simulink model "propulsionMotorPrueba"  (R2016b)
settings: Solver=VariableStepAuto  StartTime=0.0  StopTime=10.0  RelTol=1e-3
undefined symbols (not defined in the file): LD, vms
libraries: simulink x1
settings Model: Creator=Uxío  LastModifiedBy=Uxío

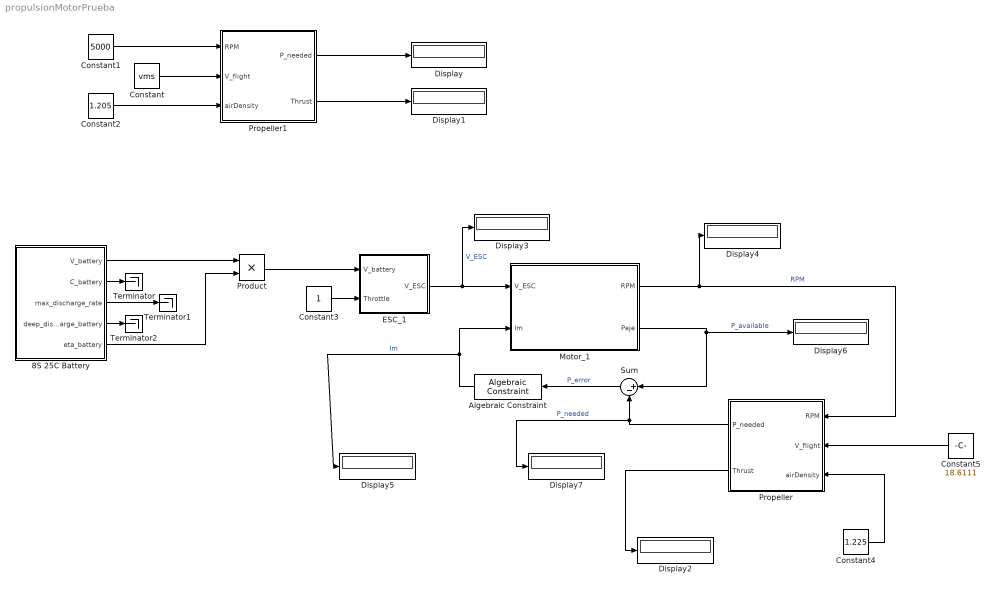
== system propulsionMotorPrueba ==
  8S 25C Battery : Subsystem
  Algebraic Constraint : simulink/Math Operations/Algebraic Constraint  z0=0
  Constant : Constant  Value=vms
  Constant1 : Constant  Value=5000
  Constant2 : Constant  Value=1.205
  Constant3 : Constant
  Constant4 : Constant  Value=1.225
  Constant5 : Constant  Value=18.6111
  Display{,1..7} (8 alike) : Display
  ESC_1 : Subsystem
  Motor_1 : Subsystem
  Product : Product
  Propeller : Subsystem
  Propeller1 : Subsystem
  Sum : Sum  Inputs=|+-
  Terminator : Terminator
  Terminator1 : Terminator
  Terminator2 : Terminator
  wires:
  Constant/1 -> Propeller1/2(V_flight)
  Constant1/1 -> Propeller1/1(RPM)
  Constant2/1 -> Propeller1/3(airDensity)
  Propeller1/1(P_needed) -> Display/1
  Propeller1/2(Thrust) -> Display1/1
  Constant3/1 -> ESC_1/2(Throttle)
  8S 25C Battery/1(V_battery) -> Product/1
  Product/1 -> ESC_1/1(V_battery)
  8S 25C Battery/5(eta_battery) -> Product/2
  8S 25C Battery/2(C_battery) -> Terminator/1
  8S 25C Battery/3(max_discharge_rate) -> Terminator1/1
  8S 25C Battery/4(deep_discharge_battery) -> Terminator2/1
  ESC_1/1(V_ESC) -> Motor_1/1(V_ESC), Display3/1  "V_ESC"
  Motor_1/1(RPM) -> Display4/1, Propeller/1(RPM)  "RPM"
  Constant5/1 -> Propeller/2(V_flight)
  Constant4/1 -> Propeller/3(airDensity)
  Propeller/1(P_needed) -> Display7/1, Sum/2  "P_needed"
  Motor_1/2(Peje) -> Display6/1, Sum/1  "P_available"
  Sum/1 -> Algebraic Constraint/1  "P_error"
  Algebraic Constraint/1 -> Motor_1/2(Im), Display5/1  "Im"
  Propeller/2(Thrust) -> Display2/1

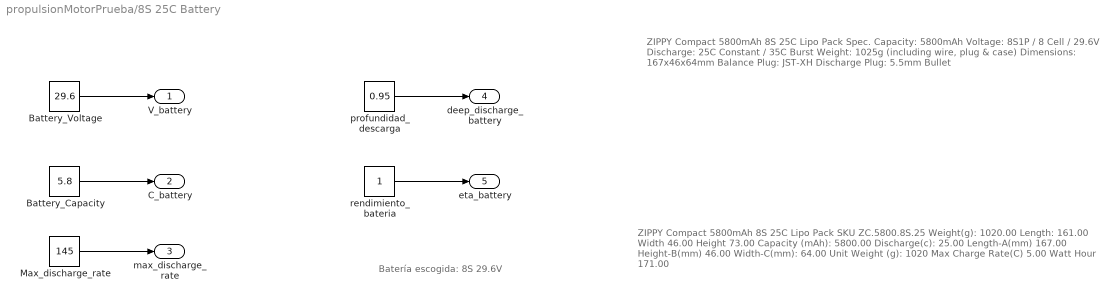
== system propulsionMotorPrueba/8S 25C Battery ==
  note: ZIPPY Compact 5800mAh 8S 25C Lipo Pack
      |
      | Spec.
      | Capacity: 5800mAh
      | Voltage: 8S1P / 8 Cell / 29.6V
      | Discharge: 25C Constant / 35C Burst
      | Weight: 1025g (including wire, plug & case)
      | Dimensions: 167x46x64mm
      | Balance Plug: JST-XH
      | Discharge Plug: 5.5mm Bullet
  note: ZIPPY Compact 5800mAh 8S 25C Lipo Pack
      |
      | SKU
      | ZC.5800.8S.25
      | Weight(g):
      | 1020.00
      | Length:
      | 161.00
      | Width
      | 46.00
      | Height
      | 73.00
      | Capacity (mAh):
      | 5800.00
      | Discharge(c):
      | 25.00
      | Length-A(mm)
      | 167.00
      | Height-B(mm)
      | 46.00
      | Width-C(mm):
      | 64.00
      | Unit Weight (g):
      | 1020
      | Max Charge Rate(C)
      | 5.00
      | Watt Hour
      | 171.00
  note: Batería escogida: 8S 29.6V
  Battery_Capacity : Constant  Value=5.8
  Battery_Voltage : Constant  Value=29.6
  Max_discharge_rate : Constant  Value=145
  profundidad_descarga : Constant  Value=0.95
  rendimiento_bateria : Constant
  V_battery : Outport  Unit=V
  C_battery : Outport  Port=2  Unit=A*h
  max_discharge_rate : Outport  Port=3  Unit=A*h
  deep_discharge_battery : Outport  Port=4  Unit=1
  eta_battery : Outport  Port=5  Unit=1
  wires:
  Battery_Voltage/1 -> V_battery/1
  Battery_Capacity/1 -> C_battery/1
  profundidad_descarga/1 -> deep_discharge_battery/1
  rendimiento_bateria/1 -> eta_battery/1
  Max_discharge_rate/1 -> max_discharge_rate/1

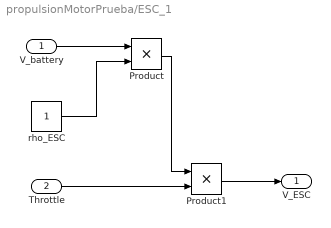
== system propulsionMotorPrueba/ESC_1 ==
  V_battery : Inport  Unit=V
  Throttle : Inport  Port=2  Unit=1
  Product : Product
  Product1 : Product
  rho_ESC : Constant
  V_ESC : Outport  Unit=V
  wires:
  rho_ESC/1 -> Product/2
  V_battery/1 -> Product/1
  Throttle/1 -> Product1/2
  Product/1 -> Product1/1
  Product1/1 -> V_ESC/1

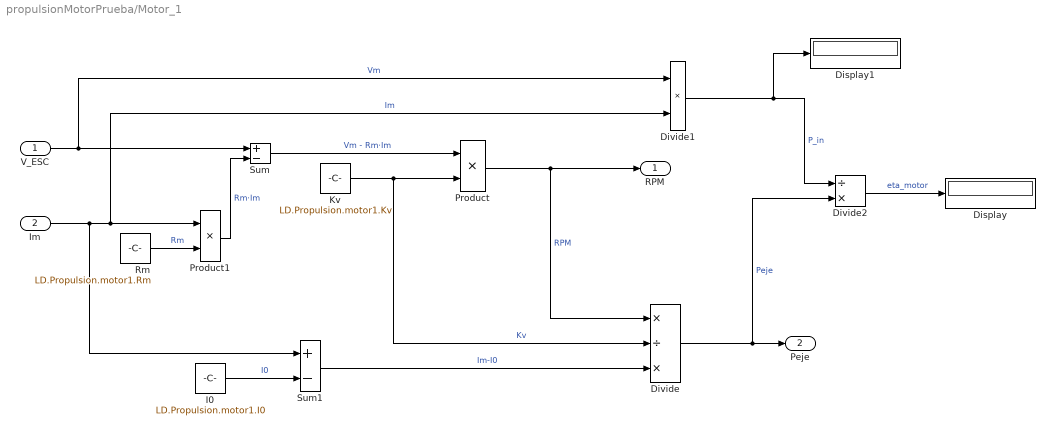
== system propulsionMotorPrueba/Motor_1 ==
  V_ESC : Inport
  Im : Inport  Port=2
  Display : Display
  Display1 : Display
  Divide : Product  Inputs=*/*
  Divide1 : Product  Inputs=**
  Divide2 : Product  Inputs=/*
  I0 : Constant  Value=LD.Propulsion.motor1.I0
  Kv : Constant  Value=LD.Propulsion.motor1.Kv
  Product : Product
  Product1 : Product
  Rm : Constant  Value=LD.Propulsion.motor1.Rm
  Sum : Sum  Inputs=+-
  Sum1 : Sum  Inputs=+-
  RPM : Outport
  Peje : Outport  Port=2
  wires:
  I0/1 -> Sum1/2  "I0"
  Kv/1 -> Divide/2, Product/2  "Kv"
  V_ESC/1 -> Divide1/1, Sum/1  "Vm"
  Rm/1 -> Product1/2  "Rm"
  Product1/1 -> Sum/2  "Rm·Im"
  Product/1 -> Divide/1, RPM/1  "RPM"
  Sum/1 -> Product/1  "Vm - Rm·Im"
  Im/1 -> Sum1/1, Divide1/2, Product1/1  "Im"
  Divide/1 -> Divide2/2, Peje/1  "Peje"
  Sum1/1 -> Divide/3  "Im-I0"
  Divide1/1 -> Display1/1, Divide2/1  "P_in"
  Divide2/1 -> Display/1  "eta_motor"

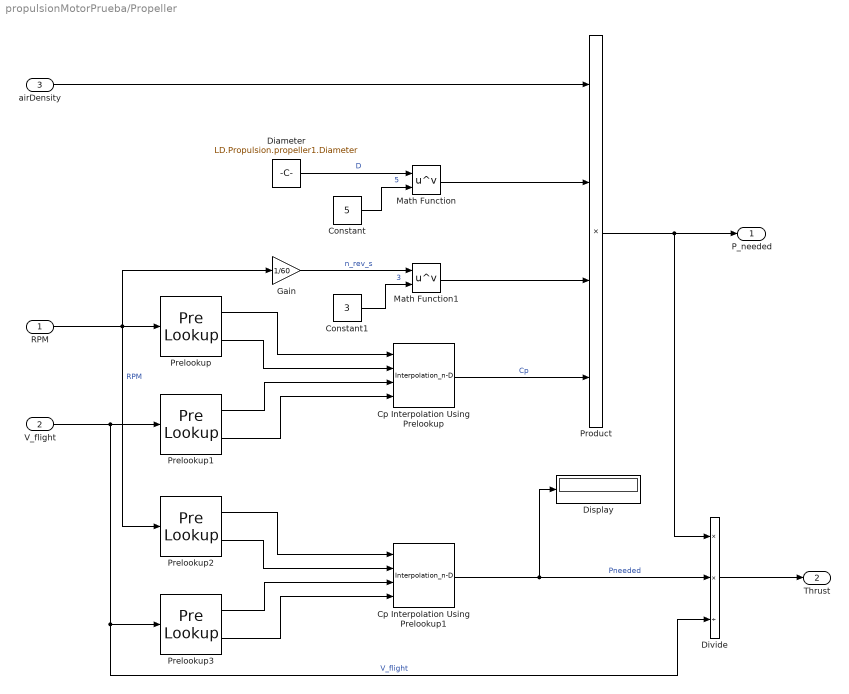
== system propulsionMotorPrueba/Propeller ==
  RPM : Inport
  V_flight : Inport  Port=2
  airDensity : Inport  Port=3
  Constant : Constant  Value=5
  Constant1 : Constant  Value=3
  Cp Interpolation Using Prelookup : Interpolation_n-D  Table=LD.Propulsion.propeller1.Cp  InternalRulePriority=Speed
  Cp Interpolation Using Prelookup1 : Interpolation_n-D  Table=LD.Propulsion.propeller1.eta  InternalRulePriority=Speed
  Diameter : Constant  Value=LD.Propulsion.propeller1.Diameter
  Display : Display
  Divide : Product  Inputs=**/
  Gain : Gain  Gain=1/60
  Math Function : Math  Operator=pow  SaturateOnIntegerOverflow=on
  Math Function1 : Math  Operator=pow  SaturateOnIntegerOverflow=on
  Prelookup : PreLookup  BreakpointsData=LD.Propulsion.propeller1.RPM  ExtrapMethod=Linear
  Prelookup1 : PreLookup  BreakpointsData=LD.Propulsion.propeller1.V  ExtrapMethod=Linear
  Prelookup2 : PreLookup  BreakpointsData=LD.Propulsion.propeller1.RPM  ExtrapMethod=Linear
  Prelookup3 : PreLookup  BreakpointsData=LD.Propulsion.propeller1.V  ExtrapMethod=Linear
  Product : Product  Inputs=4
  P_needed : Outport
  Thrust : Outport  Port=2
  wires:
  RPM/1 -> Gain/1, Prelookup/1, Prelookup2/1  "RPM"
  V_flight/1 -> Divide/3, Prelookup3/1, Prelookup1/1  "V_flight"
  Prelookup/1 -> Cp Interpolation Using Prelookup/1
  Prelookup/2 -> Cp Interpolation Using Prelookup/2
  Prelookup1/1 -> Cp Interpolation Using Prelookup/3
  Prelookup1/2 -> Cp Interpolation Using Prelookup/4
  Diameter/1 -> Math Function/1  "D"
  Constant/1 -> Math Function/2  "5"
  Constant1/1 -> Math Function1/2  "3"
  Gain/1 -> Math Function1/1  "n_rev_s"
  Cp Interpolation Using Prelookup/1 -> Product/4  "Cp"
  Math Function1/1 -> Product/3
  Math Function/1 -> Product/2
  airDensity/1 -> Product/1
  Product/1 -> Divide/1, P_needed/1
  Prelookup2/1 -> Cp Interpolation Using Prelookup1/1
  Prelookup2/2 -> Cp Interpolation Using Prelookup1/2
  Prelookup3/1 -> Cp Interpolation Using Prelookup1/3
  Prelookup3/2 -> Cp Interpolation Using Prelookup1/4
  Cp Interpolation Using Prelookup1/1 -> Display/1, Divide/2  "Pneeded"
  Divide/1 -> Thrust/1

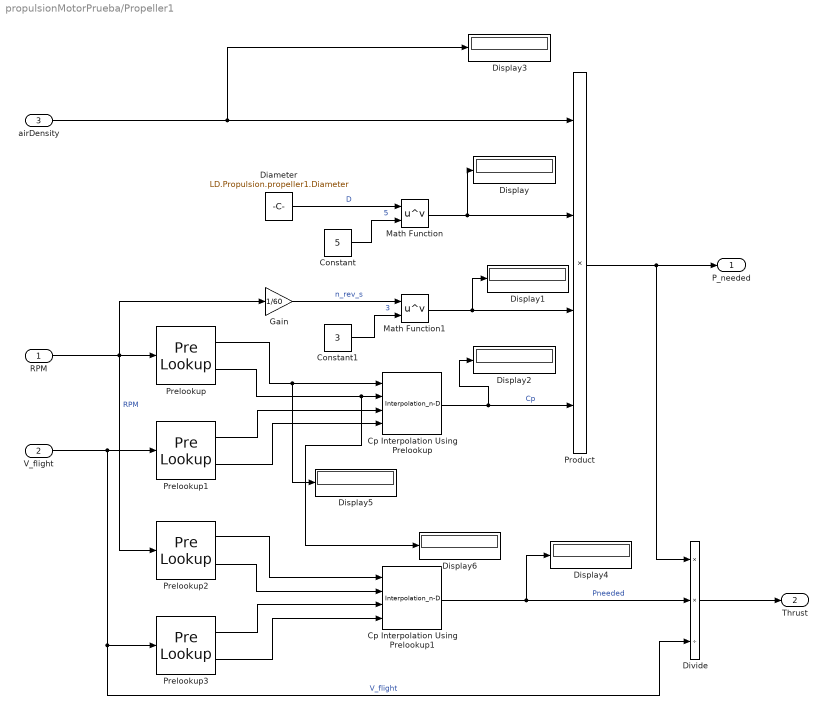
== system propulsionMotorPrueba/Propeller1 ==
  RPM : Inport
  V_flight : Inport  Port=2
  airDensity : Inport  Port=3
  Constant : Constant  Value=5
  Constant1 : Constant  Value=3
  Cp Interpolation Using Prelookup : Interpolation_n-D  Table=LD.Propulsion.propeller1.Cp  InternalRulePriority=Speed
  Cp Interpolation Using Prelookup1 : Interpolation_n-D  Table=LD.Propulsion.propeller1.eta  InternalRulePriority=Speed
  Diameter : Constant  Value=LD.Propulsion.propeller1.Diameter
  Display{,1..6} (7 alike) : Display
  Divide : Product  Inputs=**/
  Gain : Gain  Gain=1/60
  Math Function : Math  Operator=pow  SaturateOnIntegerOverflow=on
  Math Function1 : Math  Operator=pow  SaturateOnIntegerOverflow=on
  Prelookup : PreLookup  BreakpointsData=LD.Propulsion.propeller1.RPM  ExtrapMethod=Linear
  Prelookup1 : PreLookup  BreakpointsData=LD.Propulsion.propeller1.V  ExtrapMethod=Linear
  Prelookup2 : PreLookup  BreakpointsData=LD.Propulsion.propeller1.RPM  ExtrapMethod=Linear
  Prelookup3 : PreLookup  BreakpointsData=LD.Propulsion.propeller1.V  ExtrapMethod=Linear
  Product : Product  Inputs=4
  P_needed : Outport
  Thrust : Outport  Port=2
  wires:
  RPM/1 -> Gain/1, Prelookup/1, Prelookup2/1  "RPM"
  V_flight/1 -> Divide/3, Prelookup3/1, Prelookup1/1  "V_flight"
  Prelookup/1 -> Display5/1, Cp Interpolation Using Prelookup/1
  Prelookup/2 -> Display6/1, Cp Interpolation Using Prelookup/2
  Prelookup1/1 -> Cp Interpolation Using Prelookup/3
  Prelookup1/2 -> Cp Interpolation Using Prelookup/4
  Diameter/1 -> Math Function/1  "D"
  Constant/1 -> Math Function/2  "5"
  Constant1/1 -> Math Function1/2  "3"
  Gain/1 -> Math Function1/1  "n_rev_s"
  Cp Interpolation Using Prelookup/1 -> Display2/1, Product/4  "Cp"
  Math Function1/1 -> Display1/1, Product/3
  Math Function/1 -> Display/1, Product/2
  airDensity/1 -> Display3/1, Product/1
  Product/1 -> Divide/1, P_needed/1
  Prelookup2/1 -> Cp Interpolation Using Prelookup1/1
  Prelookup2/2 -> Cp Interpolation Using Prelookup1/2
  Prelookup3/1 -> Cp Interpolation Using Prelookup1/3
  Prelookup3/2 -> Cp Interpolation Using Prelookup1/4
  Cp Interpolation Using Prelookup1/1 -> Display4/1, Divide/2  "Pneeded"
  Divide/1 -> Thrust/1
